simulink model "wavelet_transform_simulink"  (R2018a)
settings: Solver=VariableStepAuto  StartTime=0.0  StopTime=10  RelTol=1e-3
libraries: dsparch4 x1
settings Model: Creator=Kaustubh  LastModifiedBy=Kaustubh
settings SolverCC: AutoInsertRateTranBlk=on
settings DataIOCC: LimitDataPoints=on  SaveOutput=off  SignalLogging=off  SaveTime=off
settings OptimizationCC: LifeSpan=inf  SimCompilerOptimization=on
settings DebuggingCC: AlgebraicLoopMsg=error  SingleTaskRateTransMsg=error  AllowSymbolicDim=off  SFUnexpectedBacktrackingDiag=warning  SFNoUnconditionalDefaultTransitionDiag=warning  SFExecutionAtInitializationDiag=none
settings CodeAppCC: StateflowObjectComments=on
settings GRTTargetCC: TargetLangStandard=C89/C90 (ANSI)  GeneratePreprocessorConditionals=Disable all
settings ConfigComp: CovMetricSettings=dw  CovHtmlReporting=on  CovSaveCumulativeToWorkspaceVar=on  CovSaveSingleToWorkspaceVar=on  CovShowResultsExplorer=off  CovExternalEMLEnable=off  CovSFcnEnable=off

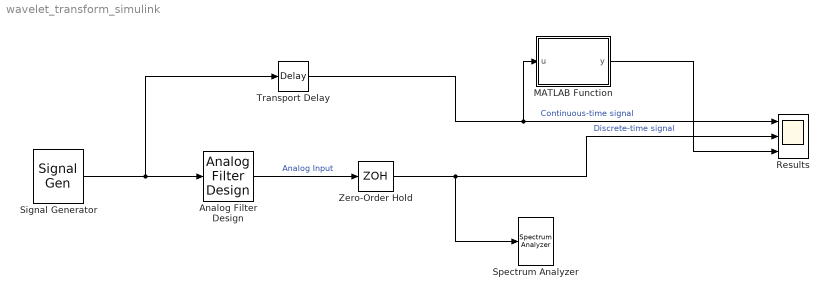
== system wavelet_transform_simulink ==
  Analog Filter Design : dsparch4/Analog Filter Design  method=Butterworth  filttype=Lowpass  N=8  Wlo=2*pi*3200  Whi=80  Rp=1  Rs=80
  MATLAB Function : MATLAB Function  TreatAsAtomicUnit=on
  Results : Scope  NumInputPorts=3
  Signal Generator : SignalGenerator  Frequency=250
  Spectrum Analyzer : SpectrumAnalyzer
  Transport Delay : TransportDelay  DelayTime=0.3e-3
  Zero-Order Hold : ZeroOrderHold  SampleTime=1/8000
  wires:
  Analog Filter Design/1 -> Zero-Order Hold/1  "Analog Input"
  Signal Generator/1 -> Analog Filter Design/1, Transport Delay/1
  Zero-Order Hold/1 -> Spectrum Analyzer/1, Results/2  "Discrete-time signal"
  Transport Delay/1 -> MATLAB Function/1(u), Results/1  "Continuous-time signal"
  MATLAB Function/1(y) -> Results/3

== matlab function wavelet_transform_simulink/MATLAB Function ==
  data: u input; y output
function y = fcn(u)
    fb = cwtfilterbank;
    [y] = cwt(u,'FilterBank',fb);
y = u;
